simulink model "Problem2"  (R2020b)
settings: Solver=VariableStepAuto  StartTime=0.0  StopTime=inf  RelTol=1e-3
settings Model: Creator=Dell  LastModifiedBy=Dell

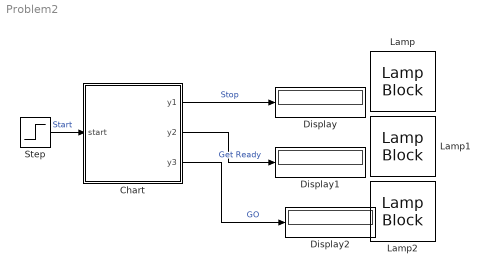
== system Problem2 ==
  Chart : Stateflow chart  TreatAsAtomicUnit=on
  Display : Display
  Display1 : Display
  Display2 : Display
  Lamp : LampBlock
  Lamp1 : LampBlock
  Lamp2 : LampBlock
  Step : Step  Time=4  SampleTime=0
  wires:
  Step/1 -> Chart/1(start)  "Start"
  Chart/1(y1) -> Display/1  "Stop"
  Chart/2(y2) -> Display1/1  "Get Ready"
  Chart/3(y3) -> Display2/1  "GO"

== stateflow chart Problem2/Chart ==
  state Red
    during:
    y1 = 1;
    y2 = 0;
    y3 = 0;
    forward = 1;
  state Yellow
    during:
    y1 = 0;
    y2 = 1;
    y3 = 0;
  state Stand_By_
    during:
    y1 = 1;
    y2 = 1;
    y3 = 1;
    forward = 0;
  state Green
    during:
    y1 = 0;
    y2 = 0;
    y3 = 1;
    forward = 0;
  Red -> Yellow : after(5,sec)[forward == 1]
  Yellow -> Green [order 1] : after(3, sec)[forward == 1]
  Yellow -> Red [order 2] : after(3, sec)[forward == 0]
  Stand_By_ -> Red : [start == 1]
  Green -> Yellow : after(5, sec)[forward == 0]
  (default) -> Stand_By_
  data: y1 output; y2 output; y3 output; forward local; start input
